simulink model "io614_can_visibility_test_R2024b"  (R2024b)
settings: Solver=FixedStepDiscrete  StartTime=0.0  StopTime=inf  FixedStep=0.001  RelTol=1e-3
values from neighbouring files (symbols this model uses):
  tx_dlc = 8    [io614_can_visibility_test_R2024b.sldd]
  tx_enable = 0    [io614_can_visibility_test_R2024b.sldd]
  tx_id = 899    [io614_can_visibility_test_R2024b.sldd]
  tx_payload_u8 : value not decoded    [io614_can_visibility_test_R2024b.sldd]
  tx_period_ms = 100.0    [io614_can_visibility_test_R2024b.sldd]
libraries: speedgoatlib_IO614 x4
settings Model: DataDictionary=io614_can_visibility_test_R2024b.sldd  Creator=aniru  LastModifiedBy=aniru
settings SolverCC: ConcurrentTasks=on  PositivePriorityOrder=on
settings OptimizationCC: BlockReduction=off  OptimizeBlockIOStorage=off
settings DebuggingCC: TasksWithSamePriorityMsg=none
settings HardwareCC: ProdBitPerLong=64  ProdLongLongMode=on  ProdHWDeviceType=Intel->x86-64 (Linux 64)
settings RTWCC: Description=Speedgoat Real-Time Target Machine  SystemTargetFile=speedgoat.tlc  TemplateMakefile=slrealtime_default_tmf  Toolchain=Simulink Real-Time Toolchain  BuildConfiguration=Faster Runs  CodeExecutionProfiling=on  TargetLang=C++
settings SimulinkRealTimeTargetCC: InstructionSetFMA=off  LogToMDFFile=off

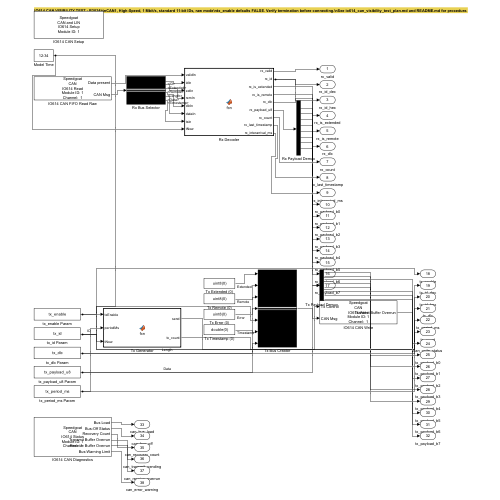
[thumbnail: Simulink's stored preview of the top-level diagram]
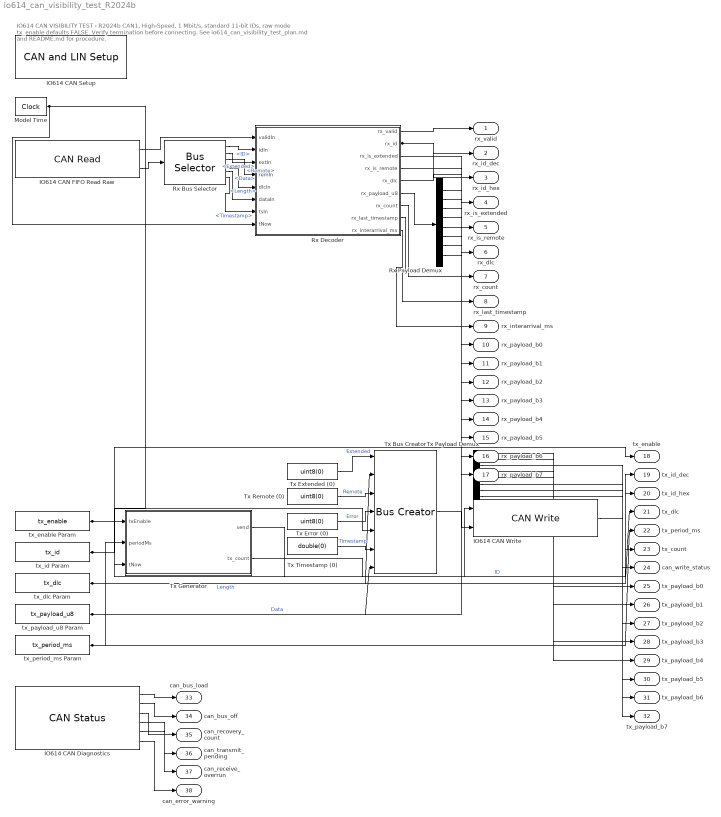
== system io614_can_visibility_test_R2024b ==
  note: IO614 CAN VISIBILITY TEST - R2024b\nCAN1, High-Speed, 1 Mbit/s, standard 11-bit IDs, raw mode\ntx_enable defaults FALSE. Verify termination before connecting.\nSee io614_can_visibility_test_plan.md and README.md for procedure.
  IO614 CAN Diagnostics : speedgoatlib_IO614/CAN Status   moduleType=IO614  id=1  channel=1  canType=CAN (HS)  autoRecovery=off  enableInput=off  ts=0.001  initValues=[614 1 0.001 0 0 0 0 0 0 0 0 0 0 0 0]
      settings: LibrarySourceBlock=speedgoatlib_CANLIN_OfA2/CAN/CAN Status
  IO614 CAN FIFO Read Raw : speedgoatlib_IO614/CAN Read   moduleType=IO614  id=1  channel=1  canType=CAN (HS)  useBusOut=on  HasMulRead=Single Read from Buffer (FIFO)  MsgIDlist=[1 2]  isEFF=off  LabelInHex=on  enableInput=off  ts=0.001  initValues=[614 1 0.001 0 1 1 0 1 0 1 2 1 2]
      settings: SourceProductName=IO614
  IO614 CAN Setup : speedgoatlib_IO614/CAN and LIN Setup   moduleInitValues="[614    1    1   -1   -1]"  id=1  moduleType=IO614  pciSlot=-1  canChn1=CAN (HS)  canChn2=Disabled  canChn3=Disabled  canChn4=Disabled  linChn1=Disabled  linChn2=Disabled  canInitStructArray=[]  canTermStructArray=[]  canChn1InitValues="[2   2   1  31   8   2   1   5   2]"  arbBdrChn1=1.0 MBaud  arbManBdrChn1=[2,1,31,8]  fdBdrChn1=5.0 MBaud  fdManBdrChn1=[2,1,5,2]  canChn2InitValues="[1   2   1  31   8   2   1   5   2]"  arbBdrChn2=1.0 MBaud  arbManBdrChn2=[2,1,31,8]  fdBdrChn2=5.0 MBaud  fdManBdrChn2=[2,1,5,2]  canChn3InitValues="[1   2   1  31   8   2   1   5   2]"  arbBdrChn3=1.0 MBaud  arbManBdrChn3=[2,1,31,8]  fdBdrChn3=5.0 MBaud  fdManBdrChn3=[2,1,5,2]  canChn4InitValues="[1   2   1  31   8   2   1   5   2]"  arbBdrChn4=1.0 MBaud  arbManBdrChn4=[2,1,31,8]  fdBdrChn4=5.0 MBaud  fdManBdrChn4=[2,1,5,2]  bdrLIN1=19200  linChn1InitValues="[1  19200]"  bdrLIN2=19200  linChn2InitValues="[1  19200]"
      settings: LibrarySourceBlock=speedgoatlib_CANLIN_OfA2/CAN and LIN Setup
  IO614 CAN Write : speedgoatlib_IO614/CAN Write   moduleType=IO614  id=1  channel=1  canType=CAN (HS)  useBusIn=on  numOfMsg=1  enableInput=on  enableStatusPort=on  initValues=[614 1 0.001 0 1 1 1 1 1 1]  ts=0.001
      settings: SourceProductName=IO614
  Model Time : DigitalClock  SampleTime=0.001
  Rx Bus Selector : BusSelector  OutputSignals=ID,Extended,Remote,Length,Data,Timestamp
  Rx Decoder : MATLAB Function  TreatAsAtomicUnit=on
  Rx Payload Demux : Demux  Outputs=8
  Tx Bus Creator : BusCreator  Inputs=7
  Tx Error (0) : Constant  Value=uint8(0)
  Tx Extended (0) : Constant  Value=uint8(0)
  Tx Generator : MATLAB Function  TreatAsAtomicUnit=on
  Tx Payload Demux : Demux  Outputs=8
  Tx Remote (0) : Constant  Value=uint8(0)
  Tx Timestamp (0) : Constant  Value=double(0)
  tx_dlc Param : Constant  Value=tx_dlc
  tx_enable Param : Constant  Value=tx_enable
  tx_id Param : Constant  Value=tx_id
  tx_payload_u8 Param : Constant  Value=tx_payload_u8
  tx_period_ms Param : Constant  Value=tx_period_ms
  rx_valid : Outport
  rx_id_dec : Outport  Port=2
  rx_id_hex : Outport  Port=3
  rx_is_extended : Outport  Port=4
  rx_is_remote : Outport  Port=5
  rx_dlc : Outport  Port=6
  rx_count : Outport  Port=7
  rx_last_timestamp : Outport  Port=8
  rx_interarrival_ms : Outport  Port=9
  rx_payload_b0 : Outport  Port=10
  rx_payload_b1 : Outport  Port=11
  rx_payload_b2 : Outport  Port=12
  rx_payload_b3 : Outport  Port=13
  rx_payload_b4 : Outport  Port=14
  rx_payload_b5 : Outport  Port=15
  rx_payload_b6 : Outport  Port=16
  rx_payload_b7 : Outport  Port=17
  tx_enable : Outport  Port=18
  tx_id_dec : Outport  Port=19
  tx_id_hex : Outport  Port=20
  tx_dlc : Outport  Port=21
  tx_period_ms : Outport  Port=22
  tx_count : Outport  Port=23
  can_write_status : Outport  Port=24
  tx_payload_b0 : Outport  Port=25
  tx_payload_b1 : Outport  Port=26
  tx_payload_b2 : Outport  Port=27
  tx_payload_b3 : Outport  Port=28
  tx_payload_b4 : Outport  Port=29
  tx_payload_b5 : Outport  Port=30
  tx_payload_b6 : Outport  Port=31
  tx_payload_b7 : Outport  Port=32
  can_bus_load : Outport  Port=33
  can_bus_off : Outport  Port=34
  can_recovery_count : Outport  Port=35
  can_transmit_pending : Outport  Port=36
  can_receive_overrun : Outport  Port=37
  can_error_warning : Outport  Port=38
  wires:
  IO614 CAN FIFO Read Raw/1 -> Rx Decoder/1(validIn)
  IO614 CAN FIFO Read Raw/2 -> Rx Bus Selector/1
  Rx Bus Selector/1 -> Rx Decoder/2(idIn)  "<ID>"
  Rx Bus Selector/2 -> Rx Decoder/3(extIn)  "<Extended>"
  Rx Bus Selector/3 -> Rx Decoder/4(remIn)  "<Remote>"
  Rx Bus Selector/4 -> Rx Decoder/5(dlcIn)  "<Length>"
  Rx Bus Selector/5 -> Rx Decoder/6(dataIn)  "<Data>"
  Rx Bus Selector/6 -> Rx Decoder/7(tsIn)  "<Timestamp>"
  Model Time/1 -> Rx Decoder/8(tNow), Tx Generator/3(tNow)
  Rx Decoder/6(rx_payload_u8) -> Rx Payload Demux/1
  Rx Decoder/1(rx_valid) -> rx_valid/1
  Rx Decoder/2(rx_id) -> rx_id_dec/1, rx_id_hex/1
  Rx Decoder/3(rx_is_extended) -> rx_is_extended/1
  Rx Decoder/4(rx_is_remote) -> rx_is_remote/1
  Rx Decoder/5(rx_dlc) -> rx_dlc/1
  Rx Decoder/7(rx_count) -> rx_count/1
  Rx Decoder/8(rx_last_timestamp) -> rx_last_timestamp/1
  Rx Decoder/9(rx_interarrival_ms) -> rx_interarrival_ms/1
  Rx Payload Demux/1 -> rx_payload_b0/1
  Rx Payload Demux/2 -> rx_payload_b1/1
  Rx Payload Demux/3 -> rx_payload_b2/1
  Rx Payload Demux/4 -> rx_payload_b3/1
  Rx Payload Demux/5 -> rx_payload_b4/1
  Rx Payload Demux/6 -> rx_payload_b5/1
  Rx Payload Demux/7 -> rx_payload_b6/1
  Rx Payload Demux/8 -> rx_payload_b7/1
  tx_enable Param/1 -> Tx Generator/1(txEnable), tx_enable/1
  tx_period_ms Param/1 -> Tx Generator/2(periodMs), tx_period_ms/1
  Tx Extended (0)/1 -> Tx Bus Creator/1  "Extended"
  tx_dlc Param/1 -> Tx Bus Creator/2, tx_dlc/1  "Length"
  Tx Remote (0)/1 -> Tx Bus Creator/3  "Remote"
  Tx Error (0)/1 -> Tx Bus Creator/4  "Error"
  tx_id Param/1 -> Tx Bus Creator/5, tx_id_dec/1, tx_id_hex/1  "ID"
  Tx Timestamp (0)/1 -> Tx Bus Creator/6  "Timestamp"
  tx_payload_u8 Param/1 -> Tx Bus Creator/7, Tx Payload Demux/1  "Data"
  Tx Generator/1(send) -> IO614 CAN Write/1
  Tx Bus Creator/1 -> IO614 CAN Write/2
  Tx Generator/2(tx_count) -> tx_count/1
  IO614 CAN Write/1 -> can_write_status/1
  Tx Payload Demux/1 -> tx_payload_b0/1
  Tx Payload Demux/2 -> tx_payload_b1/1
  Tx Payload Demux/3 -> tx_payload_b2/1
  Tx Payload Demux/4 -> tx_payload_b3/1
  Tx Payload Demux/5 -> tx_payload_b4/1
  Tx Payload Demux/6 -> tx_payload_b5/1
  Tx Payload Demux/7 -> tx_payload_b6/1
  Tx Payload Demux/8 -> tx_payload_b7/1
  IO614 CAN Diagnostics/1 -> can_bus_load/1
  IO614 CAN Diagnostics/2 -> can_bus_off/1
  IO614 CAN Diagnostics/3 -> can_recovery_count/1
  IO614 CAN Diagnostics/4 -> can_transmit_pending/1
  IO614 CAN Diagnostics/5 -> can_receive_overrun/1
  IO614 CAN Diagnostics/6 -> can_error_warning/1

== matlab function io614_can_visibility_test_R2024b/Tx Generator ==
  data: txEnable input; send output; periodMs input; tNow input; tx_count output
function [send, tx_count] = fcn(txEnable, periodMs, tNow)
%#codegen
persistent lastSendMs count
if isempty(lastSendMs)
    lastSendMs = double(-1);
    count = uint32(0);
end
nowMs = tNow * 1000;
safePeriod = max(periodMs, 1);
send = uint32(0);
if txEnable && (lastSendMs < 0 || (nowMs - lastSendMs) >= safePeriod)
    send = uint32(1);
    lastSendMs = nowMs;
    count = count + uint32(1);
end
tx_count = count;
end

== matlab function io614_can_visibility_test_R2024b/Rx Decoder ==
  data: validIn input; rx_valid output; idIn input; extIn input; remIn input; dlcIn input; dataIn input; tsIn input; tNow input; rx_id output; rx_is_extended output; rx_is_remote output; rx_dlc output; rx_payload_u8 output; rx_count output; rx_last_timestamp output; rx_interarrival_ms output
function [rx_valid, rx_id, rx_is_extended, rx_is_remote, rx_dlc, ...
    rx_payload_u8, rx_count, rx_last_timestamp, rx_interarrival_ms] = ...
    fcn(validIn, idIn, extIn, remIn, dlcIn, dataIn, tsIn, tNow)
%#codegen
persistent latchedId latchedExt latchedRem latchedDlc latchedData
persistent latchedTs count lastValidMs interarrivalMs
if isempty(latchedId)
    latchedId = uint32(0);
    latchedExt = uint8(0);
    latchedRem = uint8(0);
    latchedDlc = uint8(0);
    latchedData = uint8(zeros(1, 8));
    latchedTs = double(0);
    count = uint32(0);
    lastValidMs = double(-1);
    interarrivalMs = double(0);
end
nowMs = tNow * 1000;
if validIn
    latchedId = uint32(idIn);
    latchedExt = uint8(extIn);
    latchedRem = uint8(remIn);
    latchedDlc = uint8(dlcIn);
    latchedData = uint8(dataIn(:))';
    latchedTs = double(tsIn);
    count = count + uint32(1);
    if lastValidMs >= 0
        interarrivalMs = nowMs - lastValidMs;
    end
    lastValidMs = nowMs;
end
rx_valid = logical(validIn);
rx_id = latchedId;
rx_is_extended = latchedExt;
rx_is_remote = latchedRem;
rx_dlc = latchedDlc;
rx_payload_u8 = latchedData;
rx_count = count;
rx_last_timestamp = latchedTs;
rx_interarrival_ms = interarrivalMs;
end
